simulink library "inp"  (Simulink 7.4)
settings: Solver=ode45  StartTime=0.0  StopTime=10.0  RelTol=1e-3
undefined symbols (not defined in the file): AINP_BrkPedalInterp_X_bar, C_TASK_10MS_S, ENUM_SHIFTER_D, ENUM_SHIFTER_N, ENUM_SHIFTER_P, ENUM_SHIFTER_R, KINP_BonnetCloseVehSpdThre_kph, KINP_EDUCoolantTempFilTm_s, KINP_EDUOilPressureFilTm_s, KINP_EDUOilTempFilTm_s, KINP_EDUSynchDisp_mm, KINP_EDUSynchPosnPWMDC_pct_LowerLimit, KINP_EDUSynchPosnPWMDC_pct_ovrdflg, KINP_EDUSynchPosnPWMDC_pct_ovrdval, KINP_EDUSynchPosnPWMDC_pct_UpperLimit, KINP_ShifterPosConfirmD_s, KINP_ShifterPosConfirmN_s, KINP_ShifterPosConfirmP_s, KINP_ShifterPosConfirmR_s, KINP_SingleAccPedalFltRateLim_pct, KINP_TMSpd2VehSpdSigNeg_rpm, KINP_TMSpd2VehSpdSigPos_rpm, KINP_ValidCheck_EDUSynchPosnPWMDC_dec, KINP_ValidCheck_EDUSynchPosnPWMDC_inc, KINP_ValidCheck_EDUSynchPosnPWMDC_lim, KINP_VehSpdSigKeepThres_kph, KPH2MPS, MIN2SEC, MINP_BrkPedalInterp_pct, MPS2KPH, PI, seat_version_control_block_callbacks, TIRE_RADIUS
libraries: inp_lib x166, hcu_lib x4, simulink x1
(part 5 of 9)

== system inp/INP/INP_10MS/Message (10ms) ABS_DSC_HSC_FrP03 ==
  BHAL_IN_10ms : Inport
  BSRV_In_ovrdflgs : Inport  Port=2
  BSRV_In_ovrdvals : Inport  Port=3
  VINP_DSCMsgAlive_flg : Inport  Port=4
  Bus Selector1 : BusSelector  OutputSignals=VHAL_BrakePressureValidIn_flg
  Bus Selector110 : BusSelector  OutputSignals=VSRV_BrakePressureIn_bar_ovrdflg
  Bus Selector112 : BusSelector  OutputSignals=VSRV_BrakePressureIn_bar_ovrdval
  Bus Selector25 : BusSelector  OutputSignals=VHAL_BrakePressureIn_bar
  Bus Selector4 : BusSelector  OutputSignals=VSRV_ABSDSCHSCFrP03Active_flg_ovrdflg
  Bus Selector8 : BusSelector  OutputSignals=VSRV_ABSDSCHSCFrP03Active_flg_ovrdval
  Subsys VINP_ABSDSCHSCFrP03Active_flg : inp_lib/override  SystemSampleTime=-1  cal_ovrdflg=KINP_ABSDSCHSCFrP03Active_ovrdflg  cal_ovrdval=KINP_ABSDSCHSCFrP03Active_flg_ovrdval
  Subsys VINP_BrkPedalPosn_pct : inp_lib/valid_msgactv_sat_ovrd  SystemSampleTime=-1  cal_ovrdflg=KINP_BrakePressure_bar_ovrdflg  cal_ovrdval=KINP_BrakePressure_bar_ovrdval  lim=KINP_ValidCheck_BrakePressure_lim  inc=KINP_ValidCheck_BrakePressure_inc  dec=KINP_ValidCheck_BrakePressure_dec  default=KINP_BrakePressureDefault_bar  hi=KINP_BrakePressure_bar_Max  lo=KINP_BrakePressure_bar_Min
  inputs_bus1 : BusCreator  Inputs=3
  lu1d_BrkPedalInterp : Lookup  InputValues=AINP_BrkPedalInterp_X_bar  Table=MINP_BrkPedalInterp_pct  LookUpMeth=Interpolation-Use End Values  OutDataType=sfix(16)  OutScaling=2^0
      settings: AttributesFormatString=input=%<inputvalues>\noutput=%<outputvalues>
  BINP_ABS_DSC_HSC_FrP03 : Outport  OutDataType=sfix(16)  OutScaling=2^0
  wires:
  [BSRV_In_ovrdvals] -> Bus Selector112/1
  [BSRV_In_ovrdflgs] -> Bus Selector110/1
  inputs_bus1/1 -> BINP_ABS_DSC_HSC_FrP03/1  "BINP_ABS_DSC_HSC_FrP03"
  BSRV_In_ovrdvals/1 -> [BSRV_In_ovrdvals]
  BSRV_In_ovrdflgs/1 -> [BSRV_In_ovrdflgs]
  VINP_DSCMsgAlive_flg/1 -> [VINP_DSCMsgAlive_flg]
  BHAL_IN_10ms/1 -> Bus Selector1/1, Bus Selector25/1
  [VINP_DSCMsgAlive_flg] -> [MsgAlive_flgs], Subsys VINP_ABSDSCHSCFrP03Active_flg/1  "VHAL_ABSDSCHSCFrP03Active_flg"
  [BSRV_In_ovrdflgs] -> Bus Selector4/1
  [BSRV_In_ovrdvals] -> Bus Selector8/1
  Bus Selector4/1 -> Subsys VINP_ABSDSCHSCFrP03Active_flg/2  "<VSRV_ABSDSCHSCFrP03Active_flg_ovrdflg>"
  Bus Selector8/1 -> Subsys VINP_ABSDSCHSCFrP03Active_flg/3  "<VSRV_ABSDSCHSCFrP03Active_flg_ovrdval>"
  Subsys VINP_ABSDSCHSCFrP03Active_flg/1 -> inputs_bus1/3  "VINP_ABSDSCHSCFrP03Active_flg"
  lu1d_BrkPedalInterp/1 -> inputs_bus1/1  "VINP_BrkPedalPosn_pct"
  Bus Selector25/1 -> Subsys VINP_BrkPedalPosn_pct/1  "<VHAL_BrakePressureIn_bar>"
  Bus Selector1/1 -> Subsys VINP_BrkPedalPosn_pct/2  "<VHAL_BrakePressureValidIn_flg>"
  Bus Selector110/1 -> Subsys VINP_BrkPedalPosn_pct/3  "<VSRV_BrakePressureIn_bar_ovrdflg>"
  Bus Selector112/1 -> Subsys VINP_BrkPedalPosn_pct/4  "<VSRV_BrakePressureIn_bar_ovrdval>"
  [MsgAlive_flgs] -> Subsys VINP_BrkPedalPosn_pct/5
  Subsys VINP_BrkPedalPosn_pct/1 -> lu1d_BrkPedalInterp/1  "VINP_BrakePressure_bar"
  Subsys VINP_BrkPedalPosn_pct/2 -> inputs_bus1/2  "VINP_BrkPedalPosnValid_flg"

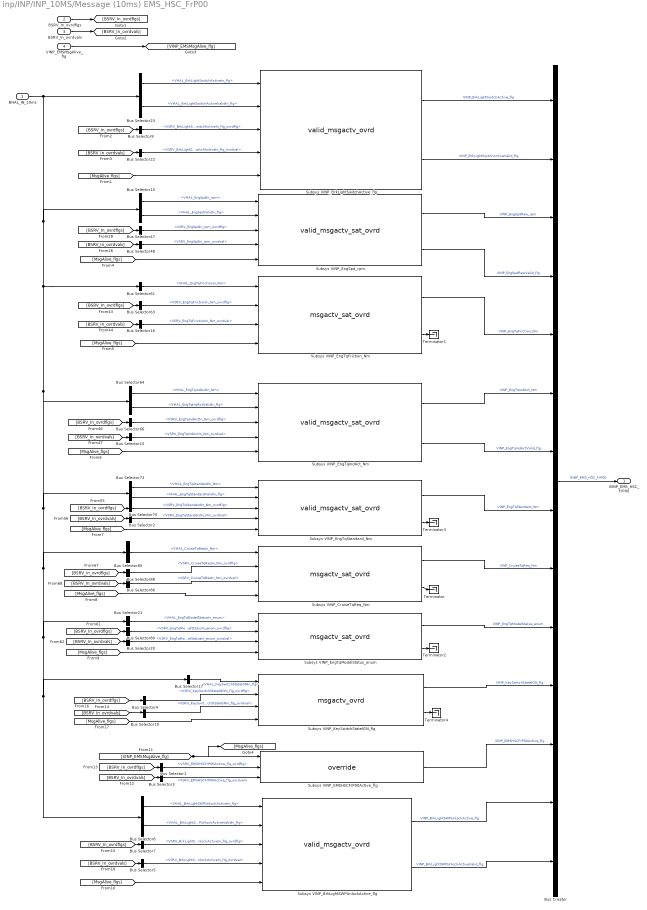
== system inp/INP/INP_10MS/Message (10ms) EMS_HSC_FrP00 ==
  BHAL_IN_10ms : Inport
  BSRV_In_ovrdflgs : Inport  Port=2
  BSRV_In_ovrdvals : Inport  Port=3
  VINP_EMSMsgAlive_flg : Inport  Port=4
  Bus Creator : BusCreator  Inputs=14
  Bus Selector1 : BusSelector  OutputSignals=VSRV_EMSHSCFrP00Active_flg_ovrdflg
  Bus Selector10 : BusSelector  OutputSignals=VHAL_EngSpdIn_rpm,VHAL_EngSpdValidIn_flg
  Bus Selector15 : BusSelector  OutputSignals=VSRV_EngTqIndActIn_Nm_ovrdval
  Bus Selector16 : BusSelector  OutputSignals=VSRV_EngTqFrictionIn_Nm_ovrdval
  Bus Selector17 : BusSelector  OutputSignals=VHAL_KeySwitchStateIGNIn_flg
  Bus Selector19 : BusSelector  OutputSignals=VSRV_KeySwitchStateIGNIn_flg_ovrdval
  Bus Selector2 : BusSelector  OutputSignals=VSRV_EngTqStandardIn_Nm_ovrdval
  Bus Selector20 : BusSelector  OutputSignals=VSRV_EngTqModelStatusIn_enum_ovrdval
  Bus Selector21 : BusSelector  OutputSignals=VHAL_EngTqModelStatusIn_enum
  Bus Selector22 : BusSelector  OutputSignals=VSRV_BrkLightSwitchActiveIn_flg_ovrdval
  Bus Selector23 : BusSelector  OutputSignals=VHAL_BrkLightSwitchActiveIn_flg,VHAL_BrkLightSwitchActiveValidIn_flg
  Bus Selector3 : BusSelector  OutputSignals=VSRV_EMSHSCFrP00Active_flg_ovrdval
  Bus Selector4 : BusSelector  OutputSignals=VSRV_KeySwitchStateIGNIn_flg_ovrdflg
  Bus Selector47 : BusSelector  OutputSignals=VSRV_EngSpdIn_rpm_ovrdflg
  Bus Selector48 : BusSelector  OutputSignals=VSRV_EngSpdIn_rpm_ovrdval
  Bus Selector5 : BusSelector  OutputSignals=VSRV_BrkLightSWPUnlockActiveIn_flg_ovrdval
  Bus Selector6 : BusSelector  OutputSignals=VHAL_BrkLightSWPUnlockActiveIn_flg,VHAL_BrkLightSWPUnlockActiveValidIn_flg
  Bus Selector61 : BusSelector  OutputSignals=VHAL_EngTqFrictionIn_Nm
  Bus Selector63 : BusSelector  OutputSignals=VSRV_EngTqFrictionIn_Nm_ovrdflg
  Bus Selector64 : BusSelector  OutputSignals=VHAL_EngTqIndActIn_Nm,VHAL_EngTqIndActValidIn_flg
  Bus Selector66 : BusSelector  OutputSignals=VSRV_EngTqIndActIn_Nm_ovrdflg
  Bus Selector7 : BusSelector  OutputSignals=VSRV_BrkLightSWPUnlockActiveIn_flg_ovrdflg
  Bus Selector73 : BusSelector  OutputSignals=VHAL_EngTqStandardIn_Nm,VHAL_EngTqStandardValidIn_flg
  Bus Selector75 : BusSelector  OutputSignals=VSRV_EngTqStandardIn_Nm_ovrdflg
  Bus Selector80 : BusSelector  OutputSignals=VSRV_EngTqModelStatusIn_enum_ovrdflg
  Bus Selector85 : BusSelector  OutputSignals=VHAL_CruiseTqReqIn_Nm
  Bus Selector86 : BusSelector  OutputSignals=VSRV_CruiseTqReqIn_Nm_ovrdval
  Bus Selector88 : BusSelector  OutputSignals=VSRV_CruiseTqReqIn_Nm_ovrdflg
  Bus Selector9 : BusSelector  OutputSignals=VSRV_BrkLightSwitchActiveIn_flg_ovrdflg
  Subsys VINP_BrkLightSWPUnlockActive_flg : inp_lib/valid_msgactv_ovrd  SystemSampleTime=-1  cal_ovrdflg=KINP_BrkLightSWPUnlockActive_flg_ovrdflg  cal_ovrdval=KINP_BrkLightSWPUnlockActive_flg_ovrdval  lim=KINP_ValidCheck_BrkLightSWPUnlockActive_lim  inc=KINP_ValidCheck_BrkLightSWPUnlockActive_inc  dec=KINP_ValidCheck_BrkLightSWPUnlockActive_dec  default=KINP_BrkLightSWPUnlockActiveDefault_flg
  Subsys VINP_BrkLightSwitchActive_flg : inp_lib/valid_msgactv_ovrd  SystemSampleTime=-1  cal_ovrdflg=KINP_BrkLightSwitchActive_flg_ovrdflg  cal_ovrdval=KINP_BrkLightSwitchActive_flg_ovrdval  lim=KINP_ValidCheck_BrkLightSwitchActive_lim  inc=KINP_ValidCheck_BrkLightSwitchActive_inc  dec=KINP_ValidCheck_BrkLightSwitchActive_dec  default=KINP_BrkLightSwitchActiveDefault_flg
  Subsys VINP_CruiseTqReq_Nm : inp_lib/msgactv_sat_ovrd  SystemSampleTime=-1  cal_ovrdflg=KINP_CruiseTqReq_Nm_ovrdflg  cal_ovrdval=KINP_CruiseTqReq_Nm_ovrdval  default=KINP_CruiseTqReqDefault_Nm  hi=KINP_CruiseTqReq_Nm_Max  lo=KINP_CruiseTqReq_Nm_Min
  Subsys VINP_EMSHSCFrP00Active_flg : inp_lib/override  SystemSampleTime=-1  cal_ovrdflg=KINP_EMSHSCFrP00Active_ovrdflg  cal_ovrdval=KINP_EMSHSCFrP00Active_flg_ovrdval
  Subsys VINP_EngSpd_rpm : inp_lib/valid_msgactv_sat_ovrd  SystemSampleTime=-1  cal_ovrdflg=KINP_EngSpd_rpm_ovrdflg  cal_ovrdval=KINP_EngSpd_rpm_ovrdval  lim=KINP_ValidCheck_EngSpd_lim  inc=KINP_ValidCheck_EngSpd_inc  dec=KINP_ValidCheck_EngSpd_dec  default=KINP_EngSpdDefault_rpm  hi=KINP_EngSpd_rpm_Max  lo=KINP_EngSpd_rpm_Min
  Subsys VINP_EngTqFriction_Nm : inp_lib/msgactv_sat_ovrd  SystemSampleTime=-1  cal_ovrdflg=KINP_EngTqFriction_Nm_ovrdflg  cal_ovrdval=KINP_EngTqFriction_Nm_ovrdval  default=KINP_EngTqFrictionDefault_Nm  hi=KINP_EngTqFriction_Nm_Max  lo=KINP_EngTqFriction_Nm_Min
  Subsys VINP_EngTqIndAct_Nm : inp_lib/valid_msgactv_sat_ovrd  SystemSampleTime=-1  cal_ovrdflg=KINP_EngTqIndAct_Nm_ovrdflg  cal_ovrdval=KINP_EngTqIndAct_Nm_ovrdval  lim=KINP_ValidCheck_EngTqIndAct_lim  inc=KINP_ValidCheck_EngTqIndAct_inc  dec=KINP_ValidCheck_EngTqIndAct_dec  default=KINP_EngTqIndActDefault_Nm  hi=KINP_EngTqIndAct_Nm_Max  lo=KINP_EngTqIndAct_Nm_Min
  Subsys VINP_EngTqModelStatus_enum : inp_lib/msgactv_sat_ovrd  SystemSampleTime=-1  cal_ovrdflg=KINP_EngTqModelStatus_enum_ovrdflg  cal_ovrdval=KINP_EngTqModelStatus_enum_ovrdval  default=KINP_EngTqModelStatusDefault_enum  hi=KINP_EngTqModelStatus_enum_Max  lo=KINP_EngTqModelStatus_enum_Min
  Subsys VINP_EngTqStandard_Nm : inp_lib/valid_msgactv_sat_ovrd  SystemSampleTime=-1  cal_ovrdflg=KINP_EngTqStandard_Nm_ovrdflg  cal_ovrdval=KINP_EngTqStandard_Nm_ovrdval  lim=KINP_ValidCheck_EngTqStandard_lim  inc=KINP_ValidCheck_EngTqStandard_inc  dec=KINP_ValidCheck_EngTqStandard_dec  default=KINP_EngTqStandardDefault_Nm  hi=KINP_EngTqStandard_Nm_Max  lo=KINP_EngTqStandard_Nm_Min
  Subsys VINP_KeySwitchStateIGN_flg : inp_lib/msgactv_ovrd  SystemSampleTime=-1  cal_ovrdflg=KINP_KeySwitchStateIGN_flg_ovrdflg  cal_ovrdval=KINP_KeySwitchStateIGN_flg_ovrdval  default=KINP_KeySwitchStateIGNDefault_flg
  Terminator{,1..4} (5 alike) : Terminator
  BINP_EMS_HSC_FrP00 : Outport  OutDataType=sfix(16)  OutScaling=2^0
  wires:
  Subsys VINP_BrkLightSwitchActive_flg/1 -> Bus Creator/1  "VINP_BrkLightSwitchActive_flg"
  Bus Selector9/1 -> Subsys VINP_BrkLightSwitchActive_flg/3  "<VSRV_BrkLightSwitchActiveIn_flg_ovrdflg>"
  Bus Selector6/2 -> Subsys VINP_BrkLightSWPUnlockActive_flg/2  "<VHAL_BrkLightSWPUnlockActiveValidIn_flg>"
  Bus Selector23/2 -> Subsys VINP_BrkLightSwitchActive_flg/2  "<VHAL_BrkLightSwitchActiveValidIn_flg>"
  [MsgAlive_flgs] -> Subsys VINP_BrkLightSwitchActive_flg/5
  Bus Selector22/1 -> Subsys VINP_BrkLightSwitchActive_flg/4  "<VSRV_BrkLightSwitchActiveIn_flg_ovrdval>"
  [VINP_EMSMsgAlive_flg] -> [MsgAlive_flgs], Subsys VINP_EMSHSCFrP00Active_flg/1
  [BSRV_In_ovrdflgs] -> Bus Selector1/1
  [BSRV_In_ovrdvals] -> Bus Selector3/1
  [BSRV_In_ovrdflgs] -> Bus Selector4/1
  [BSRV_In_ovrdvals] -> Bus Selector19/1
  VINP_EMSMsgAlive_flg/1 -> [VINP_EMSMsgAlive_flg]
  BSRV_In_ovrdflgs/1 -> [BSRV_In_ovrdflgs]
  BSRV_In_ovrdvals/1 -> [BSRV_In_ovrdvals]
  [BSRV_In_ovrdflgs] -> Bus Selector80/1
  [BSRV_In_ovrdvals] -> Bus Selector20/1
  Bus Creator/1 -> BINP_EMS_HSC_FrP00/1  "BINP_EMS_HSC_FrP00"
  [BSRV_In_ovrdflgs] -> Bus Selector9/1
  [BSRV_In_ovrdvals] -> Bus Selector22/1
  [BSRV_In_ovrdflgs] -> Bus Selector47/1
  [BSRV_In_ovrdvals] -> Bus Selector48/1
  [BSRV_In_ovrdflgs] -> Bus Selector63/1
  [BSRV_In_ovrdvals] -> Bus Selector16/1
  [BSRV_In_ovrdflgs] -> Bus Selector66/1
  [BSRV_In_ovrdvals] -> Bus Selector15/1
  [BSRV_In_ovrdflgs] -> Bus Selector75/1
  [BSRV_In_ovrdvals] -> Bus Selector2/1
  [BSRV_In_ovrdflgs] -> Bus Selector88/1
  [BSRV_In_ovrdvals] -> Bus Selector86/1
  BHAL_IN_10ms/1 -> Bus Selector61/1, Bus Selector64/1, Bus Selector73/1, Bus Selector85/1, Bus Selector21/1, Bus Selector17/1, Bus Selector6/1, Bus Selector10/1, Bus Selector23/1
  [BSRV_In_ovrdflgs] -> Bus Selector7/1
  [BSRV_In_ovrdvals] -> Bus Selector5/1
  Bus Selector6/1 -> Subsys VINP_BrkLightSWPUnlockActive_flg/1  "<VHAL_BrkLightSWPUnlockActiveIn_flg>"
  Bus Selector7/1 -> Subsys VINP_BrkLightSWPUnlockActive_flg/3  "<VSRV_BrkLightSWPUnlockActiveIn_flg_ovrdflg>"
  Bus Selector5/1 -> Subsys VINP_BrkLightSWPUnlockActive_flg/4  "<VSRV_BrkLightSWPUnlockActiveIn_flg_ovrdval>"
  [MsgAlive_flgs] -> Subsys VINP_BrkLightSWPUnlockActive_flg/5
  Subsys VINP_BrkLightSWPUnlockActive_flg/1 -> Bus Creator/13  "VINP_BrkLightSWPUnlockActive_flg"
  Subsys VINP_BrkLightSWPUnlockActive_flg/2 -> Bus Creator/14  "VINP_BrkLightSWPUnlockActiveValid_flg"
  Bus Selector23/1 -> Subsys VINP_BrkLightSwitchActive_flg/1  "<VHAL_BrkLightSwitchActiveIn_flg>"
  Subsys VINP_BrkLightSwitchActive_flg/2 -> Bus Creator/2  "VINP_BrkLightSwitchActiveValid_flg"
  Bus Selector85/1 -> Subsys VINP_CruiseTqReq_Nm/1  "<VHAL_CruiseTqReqIn_Nm>"
  Bus Selector88/1 -> Subsys VINP_CruiseTqReq_Nm/2  "<VSRV_CruiseTqReqIn_Nm_ovrdflg>"
  Bus Selector86/1 -> Subsys VINP_CruiseTqReq_Nm/3  "<VSRV_CruiseTqReqIn_Nm_ovrdval>"
  [MsgAlive_flgs] -> Subsys VINP_CruiseTqReq_Nm/4
  Subsys VINP_CruiseTqReq_Nm/1 -> Bus Creator/9  "VINP_CruiseTqReq_Nm"
  Subsys VINP_CruiseTqReq_Nm/2 -> Terminator/1
  Bus Selector1/1 -> Subsys VINP_EMSHSCFrP00Active_flg/2  "<VSRV_EMSHSCFrP00Active_flg_ovrdflg>"
  Bus Selector3/1 -> Subsys VINP_EMSHSCFrP00Active_flg/3  "<VSRV_EMSHSCFrP00Active_flg_ovrdval>"
  Subsys VINP_EMSHSCFrP00Active_flg/1 -> Bus Creator/12  "VINP_EMSHSCFrP00Active_flg"
  Bus Selector61/1 -> Subsys VINP_EngTqFriction_Nm/1  "<VHAL_EngTqFrictionIn_Nm>"
  Bus Selector63/1 -> Subsys VINP_EngTqFriction_Nm/2  "<VSRV_EngTqFrictionIn_Nm_ovrdflg>"
  Bus Selector16/1 -> Subsys VINP_EngTqFriction_Nm/3  "<VSRV_EngTqFrictionIn_Nm_ovrdval>"
  [MsgAlive_flgs] -> Subsys VINP_EngTqFriction_Nm/4
  Subsys VINP_EngTqFriction_Nm/1 -> Bus Creator/5  "VINP_EngTqFriction_Nm"
  Subsys VINP_EngTqFriction_Nm/2 -> Terminator1/1
  Bus Selector64/1 -> Subsys VINP_EngTqIndAct_Nm/1  "<VHAL_EngTqIndActIn_Nm>"
  Bus Selector64/2 -> Subsys VINP_EngTqIndAct_Nm/2  "<VHAL_EngTqIndActValidIn_flg>"
  Bus Selector66/1 -> Subsys VINP_EngTqIndAct_Nm/3  "<VSRV_EngTqIndActIn_Nm_ovrdflg>"
  Bus Selector15/1 -> Subsys VINP_EngTqIndAct_Nm/4  "<VSRV_EngTqIndActIn_Nm_ovrdval>"
  [MsgAlive_flgs] -> Subsys VINP_EngTqIndAct_Nm/5
  Subsys VINP_EngTqIndAct_Nm/1 -> Bus Creator/6  "VINP_EngTqIndAct_Nm"
  Subsys VINP_EngTqIndAct_Nm/2 -> Bus Creator/7  "VINP_EngTqIndActValid_flg"
  Bus Selector21/1 -> Subsys VINP_EngTqModelStatus_enum/1  "<VHAL_EngTqModelStatusIn_enum>"
  Bus Selector80/1 -> Subsys VINP_EngTqModelStatus_enum/2  "<VSRV_EngTqModelStatusIn_enum_ovrdflg>"
  Bus Selector20/1 -> Subsys VINP_EngTqModelStatus_enum/3  "<VSRV_EngTqModelStatusIn_enum_ovrdval>"
  [MsgAlive_flgs] -> Subsys VINP_EngTqModelStatus_enum/4
  Subsys VINP_EngTqModelStatus_enum/1 -> Bus Creator/10  "VINP_EngTqModelStatus_enum"
  Subsys VINP_EngTqModelStatus_enum/2 -> Terminator2/1
  Bus Selector73/1 -> Subsys VINP_EngTqStandard_Nm/1  "<VHAL_EngTqStandardIn_Nm>"
  Bus Selector73/2 -> Subsys VINP_EngTqStandard_Nm/2  "<VHAL_EngTqStandardValidIn_flg>"
  Bus Selector75/1 -> Subsys VINP_EngTqStandard_Nm/3  "<VSRV_EngTqStandardIn_Nm_ovrdflg>"
  Bus Selector2/1 -> Subsys VINP_EngTqStandard_Nm/4  "<VSRV_EngTqStandardIn_Nm_ovrdval>"
  [MsgAlive_flgs] -> Subsys VINP_EngTqStandard_Nm/5
  Subsys VINP_EngTqStandard_Nm/1 -> Bus Creator/8  "VINP_EngTqStandard_Nm"
  Subsys VINP_EngTqStandard_Nm/2 -> Terminator3/1
  Bus Selector17/1 -> Subsys VINP_KeySwitchStateIGN_flg/1  "<VHAL_KeySwitchStateIGNIn_flg>"
  Bus Selector4/1 -> Subsys VINP_KeySwitchStateIGN_flg/2  "<VSRV_KeySwitchStateIGNIn_flg_ovrdflg>"
  Bus Selector19/1 -> Subsys VINP_KeySwitchStateIGN_flg/3  "<VSRV_KeySwitchStateIGNIn_flg_ovrdval>"
  [MsgAlive_flgs] -> Subsys VINP_KeySwitchStateIGN_flg/4
  Subsys VINP_KeySwitchStateIGN_flg/1 -> Bus Creator/11  "VINP_KeySwitchStateIGN_flg"
  Subsys VINP_KeySwitchStateIGN_flg/2 -> Terminator4/1
  Bus Selector10/1 -> Subsys VINP_EngSpd_rpm/1  "<VHAL_EngSpdIn_rpm>"
  Bus Selector10/2 -> Subsys VINP_EngSpd_rpm/2  "<VHAL_EngSpdValidIn_flg>"
  Bus Selector47/1 -> Subsys VINP_EngSpd_rpm/3  "<VSRV_EngSpdIn_rpm_ovrdflg>"
  Bus Selector48/1 -> Subsys VINP_EngSpd_rpm/4  "<VSRV_EngSpdIn_rpm_ovrdval>"
  [MsgAlive_flgs] -> Subsys VINP_EngSpd_rpm/5
  Subsys VINP_EngSpd_rpm/1 -> Bus Creator/3  "VINP_EngSpdRaw_rpm"
  Subsys VINP_EngSpd_rpm/2 -> Bus Creator/4  "VINP_EngSpdRawValid_flg"

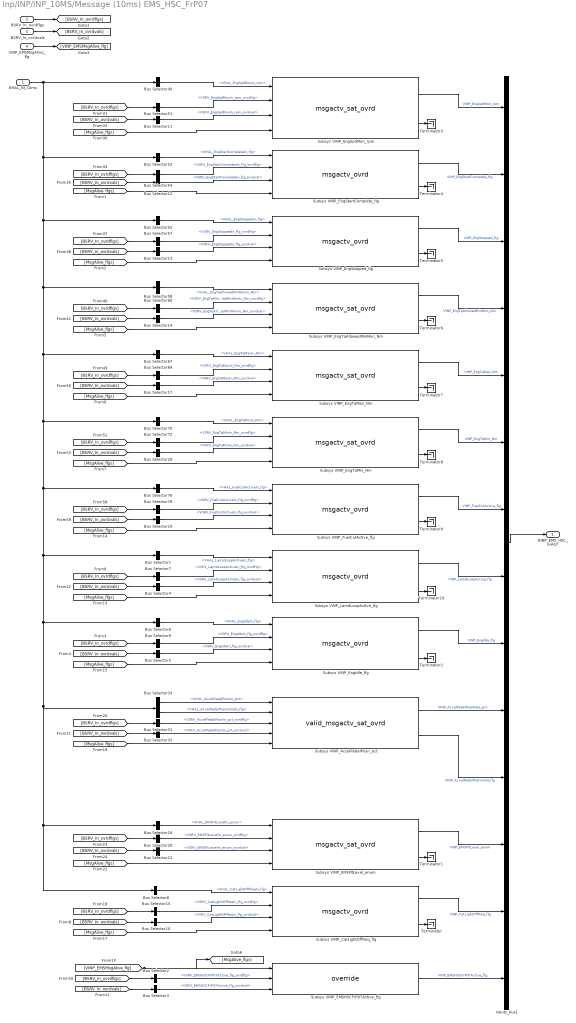
== system inp/INP/INP_10MS/Message (10ms) EMS_HSC_FrP07 ==
  BHAL_IN_10ms : Inport
  BSRV_In_ovrdflgs : Inport  Port=2
  BSRV_In_ovrdvals : Inport  Port=3
  VINP_EMSMsgAlive_flg : Inport  Port=4
  Bus Selector1 : BusSelector  OutputSignals=VHAL_LamdLoopActiveIn_flg
  Bus Selector10 : BusSelector  OutputSignals=VSRV_CatLightOffReqIn_flg_ovrdval
  Bus Selector11 : BusSelector  OutputSignals=VSRV_EngSpdMonIn_rpm_ovrdval
  Bus Selector12 : BusSelector  OutputSignals=VSRV_EngStartCompleteIn_flg_ovrdval
  Bus Selector13 : BusSelector  OutputSignals=VSRV_EngStoppedIn_flg_ovrdval
  Bus Selector14 : BusSelector  OutputSignals=VSRV_EngTqAllowedMinMonIn_Nm_ovrdval
  Bus Selector15 : BusSelector  OutputSignals=VSRV_CatLightOffReqIn_flg_ovrdflg
  Bus Selector16 : BusSelector  OutputSignals=VHAL_EMSFltLevelIn_enum
  Bus Selector17 : BusSelector  OutputSignals=VSRV_EngTqMaxIn_Nm_ovrdval
  Bus Selector18 : BusSelector  OutputSignals=VSRV_EngTqMinIn_Nm_ovrdval
  Bus Selector19 : BusSelector  OutputSignals=VSRV_FuelCutActiveIn_flg_ovrdval
  Bus Selector2 : BusSelector  OutputSignals=VSRV_EMSHSCFrP07Active_flg_ovrdflg
  Bus Selector20 : BusSelector  OutputSignals=VSRV_EMSFltLevelIn_enum_ovrdflg
  Bus Selector21 : BusSelector  OutputSignals=VSRV_EMSFltLevelIn_enum_ovrdval
  Bus Selector3 : BusSelector  OutputSignals=VSRV_EMSHSCFrP07Active_flg_ovrdval
  Bus Selector31 : BusSelector  OutputSignals=VSRV_AccelPedalPosnIn_pct_ovrdflg
  Bus Selector32 : BusSelector  OutputSignals=VSRV_AccelPedalPosnIn_pct_ovrdval
  Bus Selector33 : BusSelector  OutputSignals=VHAL_AccelPedalPosnIn_pct,VHAL_AccelPedalPosnValidIn_flg
  Bus Selector4 : BusSelector  OutputSignals=VSRV_LamdLoopActiveIn_flg_ovrdval
  Bus Selector49 : BusSelector  OutputSignals=VHAL_EngSpdMonIn_rpm
  Bus Selector5 : BusSelector  OutputSignals=VSRV_EngIdleIn_flg_ovrdval
  Bus Selector51 : BusSelector  OutputSignals=VSRV_EngSpdMonIn_rpm_ovrdflg
  Bus Selector52 : BusSelector  OutputSignals=VHAL_EngStartCompleteIn_flg
  Bus Selector54 : BusSelector  OutputSignals=VSRV_EngStartCompleteIn_flg_ovrdflg
  Bus Selector55 : BusSelector  OutputSignals=VHAL_EngStoppedIn_flg
  Bus Selector57 : BusSelector  OutputSignals=VSRV_EngStoppedIn_flg_ovrdflg
  Bus Selector58 : BusSelector  OutputSignals=VHAL_EngTqAllowedMinMonIn_Nm
  Bus Selector6 : BusSelector  OutputSignals=VHAL_EngIdleIn_flg
  Bus Selector60 : BusSelector  OutputSignals=VSRV_EngTqAllowedMinMonIn_Nm_ovrdflg
  Bus Selector67 : BusSelector  OutputSignals=VHAL_EngTqMaxIn_Nm
  Bus Selector69 : BusSelector  OutputSignals=VSRV_EngTqMaxIn_Nm_ovrdflg
  Bus Selector7 : BusSelector  OutputSignals=VSRV_LamdLoopActiveIn_flg_ovrdflg
  Bus Selector70 : BusSelector  OutputSignals=VHAL_EngTqMinIn_Nm
  Bus Selector72 : BusSelector  OutputSignals=VSRV_EngTqMinIn_Nm_ovrdflg
  Bus Selector76 : BusSelector  OutputSignals=VHAL_FuelCutActiveIn_flg
  Bus Selector78 : BusSelector  OutputSignals=VSRV_FuelCutActiveIn_flg_ovrdflg
  Bus Selector8 : BusSelector  OutputSignals=VHAL_CatLightOffReqIn_flg
  Bus Selector9 : BusSelector  OutputSignals=VSRV_EngIdleIn_flg_ovrdflg
  Subsys VINP_AccelPedalPosn_pct : inp_lib/valid_msgactv_sat_ovrd  SystemSampleTime=-1  cal_ovrdflg=KINP_AccelPedalPosn_pct_ovrdflg  cal_ovrdval=KINP_AccelPedalPosn_pct_ovrdval  lim=KINP_ValidCheck_AccelPedalPosn_lim  inc=KINP_ValidCheck_AccelPedalPosn_inc  dec=KINP_ValidCheck_AccelPedalPosn_dec  default=KINP_AccelPedalPosnDefault_pct  hi=KINP_AccelPedalPosn_pct_Max  lo=KINP_AccelPedalPosn_pct_Min
  Subsys VINP_CatLightOffReq_flg : inp_lib/msgactv_ovrd  SystemSampleTime=-1  cal_ovrdflg=KINP_CatLightOffReq_flg_ovrdflg  cal_ovrdval=KINP_CatLightOffReq_flg_ovrdval  default=KINP_CatLightOffReqDefault_flg
  Subsys VINP_EMSFltLevel_enum : inp_lib/msgactv_sat_ovrd  SystemSampleTime=-1  cal_ovrdflg=KINP_EMSFltLevel_enum_ovrdflg  cal_ovrdval=KINP_EMSFltLevel_enum_ovrdval  default=KINP_EMSFltLevelDefault_enum  hi=KINP_EMSFltLevel_enum_Max  lo=KINP_EMSFltLevel_enum_Min
  Subsys VINP_EMSHSCFrP07Active_flg : inp_lib/override  SystemSampleTime=-1  cal_ovrdflg=KINP_EMSHSCFrP07Active_ovrdflg  cal_ovrdval=KINP_EMSHSCFrP07Active_flg_ovrdval
  Subsys VINP_EngIdle_flg : inp_lib/msgactv_ovrd  SystemSampleTime=-1  cal_ovrdflg=KINP_EngIdle_flg_ovrdflg  cal_ovrdval=KINP_EngIdle_flg_ovrdval  default=KINP_EngIdleDefault_flg
  Subsys VINP_EngSpdMon_rpm : inp_lib/msgactv_sat_ovrd  SystemSampleTime=-1  cal_ovrdflg=KINP_EngSpdMon_rpm_ovrdflg  cal_ovrdval=KINP_EngSpdMon_rpm_ovrdval  default=KINP_EngSpdMonDefault_rpm  hi=KINP_EngSpdMon_rpm_Max  lo=KINP_EngSpdMon_rpm_Min
  Subsys VINP_EngStartComplete_flg : inp_lib/msgactv_ovrd  SystemSampleTime=-1  cal_ovrdflg=KINP_EngStartComplete_flg_ovrdflg  cal_ovrdval=KINP_EngStartComplete_flg_ovrdval  default=KINP_EngStartCompleteDefault_flg
  Subsys VINP_EngStopped_flg : inp_lib/msgactv_ovrd  SystemSampleTime=-1  cal_ovrdflg=KINP_EngStopped_flg_ovrdflg  cal_ovrdval=KINP_EngStopped_flg_ovrdval  default=KINP_EngStoppedDefault_flg
  Subsys VINP_EngTqAllowedMinMon_Nm : inp_lib/msgactv_sat_ovrd  SystemSampleTime=-1  cal_ovrdflg=KINP_EngTqAllowedMinMon_Nm_ovrdflg  cal_ovrdval=KINP_EngTqAllowedMinMon_Nm_ovrdval  default=KINP_EngTqAllowedMinMonDefault_Nm  hi=KINP_EngTqAllowedMinMon_Nm_Max  lo=KINP_EngTqAllowedMinMon_Nm_Min
  Subsys VINP_EngTqMax_Nm : inp_lib/msgactv_sat_ovrd  SystemSampleTime=-1  cal_ovrdflg=KINP_EngTqMax_Nm_ovrdflg  cal_ovrdval=KINP_EngTqMax_Nm_ovrdval  default=KINP_EngTqMaxDefault_Nm  hi=KINP_EngTqMax_Nm_Max  lo=KINP_EngTqMax_Nm_Min
  Subsys VINP_EngTqMin_Nm : inp_lib/msgactv_sat_ovrd  SystemSampleTime=-1  cal_ovrdflg=KINP_EngTqMin_Nm_ovrdflg  cal_ovrdval=KINP_EngTqMin_Nm_ovrdval  default=KINP_EngTqMinDefault_Nm  hi=KINP_EngTqMin_Nm_Max  lo=KINP_EngTqMin_Nm_Min
  Subsys VINP_FuelCutActive_flg : inp_lib/msgactv_ovrd  SystemSampleTime=-1  cal_ovrdflg=KINP_FuelCutActive_flg_ovrdflg  cal_ovrdval=KINP_FuelCutActive_flg_ovrdval  default=KINP_FuelCutActiveDefault_flg
  Subsys VINP_LamdLoopActive_flg : inp_lib/msgactv_ovrd  SystemSampleTime=-1  cal_ovrdflg=KINP_LamdLoopActive_flg_ovrdflg  cal_ovrdval=KINP_LamdLoopActive_flg_ovrdval  default=KINP_LamdLoopActiveDefault_flg
  Terminator{,1..10} (11 alike) : Terminator
  inputs_bus1 : BusCreator  Inputs=14
  BINP_EMS_HSC_FrP07 : Outport  OutDataType=sfix(16)  OutScaling=2^0
  wires:
  [BSRV_In_ovrdflgs] -> Bus Selector20/1
  [BSRV_In_ovrdvals] -> Bus Selector21/1
  [BSRV_In_ovrdvals] -> Bus Selector3/1
  [BSRV_In_ovrdflgs] -> Bus Selector2/1
  [VINP_EMSMsgAlive_flg] -> [MsgAlive_flgs], Subsys VINP_EMSHSCFrP07Active_flg/1
  [BSRV_In_ovrdflgs] -> Bus Selector15/1
  [BSRV_In_ovrdvals] -> Bus Selector10/1
  [BSRV_In_ovrdvals] -> Bus Selector13/1
  [BSRV_In_ovrdflgs] -> Bus Selector57/1
  [BSRV_In_ovrdvals] -> Bus Selector5/1
  [BSRV_In_ovrdflgs] -> Bus Selector9/1
  [BSRV_In_ovrdvals] -> Bus Selector19/1
  [BSRV_In_ovrdflgs] -> Bus Selector78/1
  [BSRV_In_ovrdvals] -> Bus Selector18/1
  [BSRV_In_ovrdflgs] -> Bus Selector72/1
  [BSRV_In_ovrdvals] -> Bus Selector17/1
  [BSRV_In_ovrdflgs] -> Bus Selector69/1
  [BSRV_In_ovrdvals] -> Bus Selector14/1
  [BSRV_In_ovrdflgs] -> Bus Selector60/1
  [BSRV_In_ovrdvals] -> Bus Selector12/1
  [BSRV_In_ovrdflgs] -> Bus Selector54/1
  [BSRV_In_ovrdvals] -> Bus Selector11/1
  [BSRV_In_ovrdflgs] -> Bus Selector51/1
  BHAL_IN_10ms/1 -> Bus Selector16/1, Bus Selector8/1, Bus Selector33/1, Bus Selector6/1, Bus Selector1/1, Bus Selector76/1, Bus Selector70/1, Bus Selector67/1, Bus Selector58/1, Bus Selector55/1, Bus Selector52/1, Bus Selector49/1
  VINP_EMSMsgAlive_flg/1 -> [VINP_EMSMsgAlive_flg]
  BSRV_In_ovrdflgs/1 -> [BSRV_In_ovrdflgs]
  BSRV_In_ovrdvals/1 -> [BSRV_In_ovrdvals]
  [BSRV_In_ovrdflgs] -> Bus Selector7/1
  [BSRV_In_ovrdvals] -> Bus Selector4/1
  [BSRV_In_ovrdvals] -> Bus Selector32/1
  [BSRV_In_ovrdflgs] -> Bus Selector31/1
  inputs_bus1/1 -> BINP_EMS_HSC_FrP07/1
  Bus Selector8/1 -> Subsys VINP_CatLightOffReq_flg/1  "<VHAL_CatLightOffReqIn_flg>"
  Bus Selector15/1 -> Subsys VINP_CatLightOffReq_flg/2  "<VSRV_CatLightOffReqIn_flg_ovrdflg>"
  Bus Selector10/1 -> Subsys VINP_CatLightOffReq_flg/3  "<VSRV_CatLightOffReqIn_flg_ovrdval>"
  [MsgAlive_flgs] -> Subsys VINP_CatLightOffReq_flg/4
  Subsys VINP_CatLightOffReq_flg/1 -> inputs_bus1/13  "VINP_CatLightOffReq_flg"
  Subsys VINP_CatLightOffReq_flg/2 -> Terminator/1
  Bus Selector16/1 -> Subsys VINP_EMSFltLevel_enum/1  "<VHAL_EMSFltLevelIn_enum>"
  Bus Selector20/1 -> Subsys VINP_EMSFltLevel_enum/2  "<VSRV_EMSFltLevelIn_enum_ovrdflg>"
  Bus Selector21/1 -> Subsys VINP_EMSFltLevel_enum/3  "<VSRV_EMSFltLevelIn_enum_ovrdval>"
  [MsgAlive_flgs] -> Subsys VINP_EMSFltLevel_enum/4
  Subsys VINP_EMSFltLevel_enum/1 -> inputs_bus1/12  "VINP_EMSFltLevel_enum"
  Subsys VINP_EMSFltLevel_enum/2 -> Terminator1/1
  Bus Selector2/1 -> Subsys VINP_EMSHSCFrP07Active_flg/2  "<VSRV_EMSHSCFrP07Active_flg_ovrdflg>"
  Bus Selector3/1 -> Subsys VINP_EMSHSCFrP07Active_flg/3  "<VSRV_EMSHSCFrP07Active_flg_ovrdval>"
  Subsys VINP_EMSHSCFrP07Active_flg/1 -> inputs_bus1/14  "VINP_EMSHSCFrP07Active_flg"
  Bus Selector6/1 -> Subsys VINP_EngIdle_flg/1  "<VHAL_EngIdleIn_flg>"
  Bus Selector9/1 -> Subsys VINP_EngIdle_flg/2  "<VSRV_EngIdleIn_flg_ovrdflg>"
  Bus Selector5/1 -> Subsys VINP_EngIdle_flg/3  "<VSRV_EngIdleIn_flg_ovrdval>"
  [MsgAlive_flgs] -> Subsys VINP_EngIdle_flg/4
  Subsys VINP_EngIdle_flg/1 -> inputs_bus1/9  "VINP_EngIdle_flg"
  Subsys VINP_EngIdle_flg/2 -> Terminator2/1
  Bus Selector49/1 -> Subsys VINP_EngSpdMon_rpm/1  "<VHAL_EngSpdMonIn_rpm>"
  Bus Selector51/1 -> Subsys VINP_EngSpdMon_rpm/2  "<VSRV_EngSpdMonIn_rpm_ovrdflg>"
  Bus Selector11/1 -> Subsys VINP_EngSpdMon_rpm/3  "<VSRV_EngSpdMonIn_rpm_ovrdval>"
  [MsgAlive_flgs] -> Subsys VINP_EngSpdMon_rpm/4
  Subsys VINP_EngSpdMon_rpm/1 -> inputs_bus1/1  "VINP_EngSpdMon_rpm"
  Subsys VINP_EngSpdMon_rpm/2 -> Terminator3/1
  Bus Selector52/1 -> Subsys VINP_EngStartComplete_flg/1  "<VHAL_EngStartCompleteIn_flg>"
  Bus Selector54/1 -> Subsys VINP_EngStartComplete_flg/2  "<VSRV_EngStartCompleteIn_flg_ovrdflg>"
  Bus Selector12/1 -> Subsys VINP_EngStartComplete_flg/3  "<VSRV_EngStartCompleteIn_flg_ovrdval>"
  [MsgAlive_flgs] -> Subsys VINP_EngStartComplete_flg/4
  Subsys VINP_EngStartComplete_flg/1 -> inputs_bus1/2  "VINP_EngStartComplete_flg"
  Subsys VINP_EngStartComplete_flg/2 -> Terminator4/1
  Bus Selector55/1 -> Subsys VINP_EngStopped_flg/1  "<VHAL_EngStoppedIn_flg>"
  Bus Selector57/1 -> Subsys VINP_EngStopped_flg/2  "<VSRV_EngStoppedIn_flg_ovrdflg>"
  Bus Selector13/1 -> Subsys VINP_EngStopped_flg/3  "<VSRV_EngStoppedIn_flg_ovrdval>"
  [MsgAlive_flgs] -> Subsys VINP_EngStopped_flg/4
  Subsys VINP_EngStopped_flg/1 -> inputs_bus1/3  "VINP_EngStopped_flg"
  Subsys VINP_EngStopped_flg/2 -> Terminator5/1
  Bus Selector58/1 -> Subsys VINP_EngTqAllowedMinMon_Nm/1  "<VHAL_EngTqAllowedMinMonIn_Nm>"
  Bus Selector60/1 -> Subsys VINP_EngTqAllowedMinMon_Nm/2  "<VSRV_EngTqAllowedMinMonIn_Nm_ovrdflg>"
  Bus Selector14/1 -> Subsys VINP_EngTqAllowedMinMon_Nm/3  "<VSRV_EngTqAllowedMinMonIn_Nm_ovrdval>"
  [MsgAlive_flgs] -> Subsys VINP_EngTqAllowedMinMon_Nm/4
  Subsys VINP_EngTqAllowedMinMon_Nm/1 -> inputs_bus1/4  "VINP_EngTqAllowedMinMon_Nm"
  Subsys VINP_EngTqAllowedMinMon_Nm/2 -> Terminator6/1
  Bus Selector67/1 -> Subsys VINP_EngTqMax_Nm/1  "<VHAL_EngTqMaxIn_Nm>"
  Bus Selector69/1 -> Subsys VINP_EngTqMax_Nm/2  "<VSRV_EngTqMaxIn_Nm_ovrdflg>"
  Bus Selector17/1 -> Subsys VINP_EngTqMax_Nm/3  "<VSRV_EngTqMaxIn_Nm_ovrdval>"
  [MsgAlive_flgs] -> Subsys VINP_EngTqMax_Nm/4
  Subsys VINP_EngTqMax_Nm/1 -> inputs_bus1/5  "VINP_EngTqMax_Nm"
  Subsys VINP_EngTqMax_Nm/2 -> Terminator7/1
  Bus Selector70/1 -> Subsys VINP_EngTqMin_Nm/1  "<VHAL_EngTqMinIn_Nm>"
  Bus Selector72/1 -> Subsys VINP_EngTqMin_Nm/2  "<VSRV_EngTqMinIn_Nm_ovrdflg>"
  Bus Selector18/1 -> Subsys VINP_EngTqMin_Nm/3  "<VSRV_EngTqMinIn_Nm_ovrdval>"
  [MsgAlive_flgs] -> Subsys VINP_EngTqMin_Nm/4
  Subsys VINP_EngTqMin_Nm/1 -> inputs_bus1/6  "VINP_EngTqMin_Nm"
  Subsys VINP_EngTqMin_Nm/2 -> Terminator8/1
  Bus Selector76/1 -> Subsys VINP_FuelCutActive_flg/1  "<VHAL_FuelCutActiveIn_flg>"
  Bus Selector78/1 -> Subsys VINP_FuelCutActive_flg/2  "<VSRV_FuelCutActiveIn_flg_ovrdflg>"
  Bus Selector19/1 -> Subsys VINP_FuelCutActive_flg/3  "<VSRV_FuelCutActiveIn_flg_ovrdval>"
  [MsgAlive_flgs] -> Subsys VINP_FuelCutActive_flg/4
  Subsys VINP_FuelCutActive_flg/1 -> inputs_bus1/7  "VINP_FuelCutActive_flg"
  Subsys VINP_FuelCutActive_flg/2 -> Terminator9/1
  Bus Selector1/1 -> Subsys VINP_LamdLoopActive_flg/1  "<VHAL_LamdLoopActiveIn_flg>"
  Bus Selector7/1 -> Subsys VINP_LamdLoopActive_flg/2  "<VSRV_LamdLoopActiveIn_flg_ovrdflg>"
  Bus Selector4/1 -> Subsys VINP_LamdLoopActive_flg/3  "<VSRV_LamdLoopActiveIn_flg_ovrdval>"
  [MsgAlive_flgs] -> Subsys VINP_LamdLoopActive_flg/4
  Subsys VINP_LamdLoopActive_flg/1 -> inputs_bus1/8  "VINP_LamdLoopActive_flg"
  Subsys VINP_LamdLoopActive_flg/2 -> Terminator10/1
  Bus Selector33/1 -> Subsys VINP_AccelPedalPosn_pct/1  "<VHAL_AccelPedalPosnIn_pct>"
  Bus Selector33/2 -> Subsys VINP_AccelPedalPosn_pct/2  "<VHAL_AccelPedalPosnValidIn_flg>"
  Bus Selector31/1 -> Subsys VINP_AccelPedalPosn_pct/3  "<VSRV_AccelPedalPosnIn_pct_ovrdflg>"
  Bus Selector32/1 -> Subsys VINP_AccelPedalPosn_pct/4  "<VSRV_AccelPedalPosnIn_pct_ovrdval>"
  [MsgAlive_flgs] -> Subsys VINP_AccelPedalPosn_pct/5
  Subsys VINP_AccelPedalPosn_pct/1 -> inputs_bus1/10  "VINP_AccelPedalPosnRaw_pct"
  Subsys VINP_AccelPedalPosn_pct/2 -> inputs_bus1/11  "VINP_AccelPedalPosnValid_flg"

== system inp/INP/INP_10MS/Message (10ms) ISC_HSC2_FrP03 ==
  BHAL_IN_10ms : Inport
  BSRV_In_ovrdflgs : Inport  Port=2
  BSRV_In_ovrdvals : Inport  Port=3
  VINP_ISCMsgAlive_flg : Inport  Port=4
  Bus Creator : BusCreator  Inputs=8
  Bus Selector1 : BusSelector  OutputSignals=VSRV_ISGDiagReqIn_flg_ovrdval
  Bus Selector103 : BusSelector  OutputSignals=VHAL_ISGTqActIn_Nm
  Bus Selector104 : BusSelector  OutputSignals=VSRV_ISGTqActIn_Nm_ovrdflg
  Bus Selector16 : BusSelector  OutputSignals=VSRV_ISGACShortCircReadyIn_flg_ovrdflg
  Bus Selector17 : BusSelector  OutputSignals=VHAL_ISGACShortCircReadyIn_flg
  Bus Selector18 : BusSelector  OutputSignals=VHAL_ISGSpdIn_rpm
  Bus Selector19 : BusSelector  OutputSignals=VSRV_ISGACShortCircReadyIn_flg_ovrdval
  Bus Selector2 : BusSelector  OutputSignals=VSRV_ISCHSC2FrP03Active_flg_ovrdflg
  Bus Selector23 : BusSelector  OutputSignals=VSRV_ISGTqActIn_Nm_ovrdval
  Bus Selector3 : BusSelector  OutputSignals=VSRV_ISCHSC2FrP03Active_flg_ovrdval
  Bus Selector4 : BusSelector  OutputSignals=VHAL_ISGSpdValidIn_flg
  Bus Selector5 : BusSelector  OutputSignals=VHAL_ISGTqActValidIn_flg
  Bus Selector56 : BusSelector  OutputSignals=VHAL_ISGModeIn_enum
  Bus Selector57 : BusSelector  OutputSignals=VSRV_ISGModeIn_enum_ovrdflg
  Bus Selector6 : BusSelector  OutputSignals=VHAL_ISGDiagReqIn_flg
  Bus Selector7 : BusSelector  OutputSignals=VSRV_ISGDiagReqIn_flg_ovrdflg
  Bus Selector8 : BusSelector  OutputSignals=VSRV_ISGModeIn_enum_ovrdval
  Bus Selector86 : BusSelector  OutputSignals=VSRV_ISGSpdIn_rpm_ovrdflg
  Bus Selector87 : BusSelector  OutputSignals=VSRV_ISGSpdIn_rpm_ovrdval
  Subsys VINP_ISCHSC2FrP03Active_flg : inp_lib/override  SystemSampleTime=-1  cal_ovrdflg=KINP_ISCHSC2FrP03Active_ovrdflg  cal_ovrdval=KINP_ISCHSC2FrP03Active_flg_ovrdval
  Subsys VINP_ISGACShortCircReady_flg : inp_lib/msgactv_ovrd  SystemSampleTime=-1  cal_ovrdflg=KINP_ISGACShortCircReady_flg_ovrdflg  cal_ovrdval=KINP_ISGACShortCircReady_flg_ovrdval  default=KINP_ISGACShortCircReadyDefault_flg
  Subsys VINP_ISGDiagReq_flg : inp_lib/msgactv_ovrd  SystemSampleTime=-1  cal_ovrdflg=KINP_ISGDiagReq_flg_ovrdflg  cal_ovrdval=KINP_ISGDiagReq_flg_ovrdval  default=KINP_ISGDiagReqDefault_flg
  Subsys VINP_ISGMode_enum : inp_lib/msgactv_sat_ovrd  SystemSampleTime=-1  cal_ovrdflg=KINP_ISGMode_enum_ovrdflg  cal_ovrdval=KINP_ISGMode_enum_ovrdval  default=KINP_ISGModeDefault_enum  hi=KINP_ISGMode_enum_Max  lo=KINP_ISGMode_enum_Min
  Subsys VINP_ISGSpeed_rpm : inp_lib/valid_msgactv_sat_ovrd  SystemSampleTime=-1  cal_ovrdflg=KINP_ISGSpd_rpm_ovrdflg  cal_ovrdval=KINP_ISGSpd_rpm_ovrdval  lim=KINP_ValidCheck_ISGSpd_lim  inc=KINP_ValidCheck_ISGSpd_inc  dec=KINP_ValidCheck_ISGSpd_dec  default=KINP_ISGSpdDefault_rpm  hi=KINP_ISGSpd_rpm_Max  lo=KINP_ISGSpd_rpm_Min
  Subsys VINP_ISGTqAct_Nm : inp_lib/valid_msgactv_sat_ovrd  SystemSampleTime=-1  cal_ovrdflg=KINP_ISGTqAct_Nm_ovrdflg  cal_ovrdval=KINP_ISGTqAct_Nm_ovrdval  lim=KINP_ValidCheck_ISGTqAct_lim  inc=KINP_ValidCheck_ISGTqAct_inc  dec=KINP_ValidCheck_ISGTqAct_dec  default=KINP_ISGTqActDefault_Nm  hi=KINP_ISGTqAct_Nm_Max  lo=KINP_ISGTqAct_Nm_Min
  Terminator : Terminator
  Terminator1 : Terminator
  Terminator2 : Terminator
  BINP_ISC_HSC2_FrP03 : Outport
  wires:
  Bus Creator/1 -> BINP_ISC_HSC2_FrP03/1  "BINP_ISC_HSC2_FrP03"
  BSRV_In_ovrdvals/1 -> [BSRV_In_ovrdvals]
  BSRV_In_ovrdflgs/1 -> [BSRV_In_ovrdflgs]
  VINP_ISCMsgAlive_flg/1 -> [VINP_ISCMsgAlive_flg]
  [BSRV_In_ovrdflgs] -> Bus Selector16/1
  [BSRV_In_ovrdvals] -> Bus Selector19/1
  BHAL_IN_10ms/1 -> Bus Selector6/1, Bus Selector56/1, Bus Selector18/1, Bus Selector4/1, Bus Selector103/1, Bus Selector5/1, Bus Selector17/1
  [VINP_ISCMsgAlive_flg] -> [MsgAlive_flgs], Subsys VINP_ISCHSC2FrP03Active_flg/1  "VHAL_ISCHSC2FrP03Active_flg"
  [BSRV_In_ovrdflgs] -> Bus Selector2/1
  [BSRV_In_ovrdvals] -> Bus Selector3/1
  [BSRV_In_ovrdflgs] -> Bus Selector7/1
  [BSRV_In_ovrdvals] -> Bus Selector1/1
  [BSRV_In_ovrdvals] -> Bus Selector23/1
  [BSRV_In_ovrdflgs] -> Bus Selector104/1
  [BSRV_In_ovrdvals] -> Bus Selector87/1
  [BSRV_In_ovrdflgs] -> Bus Selector86/1
  [BSRV_In_ovrdflgs] -> Bus Selector57/1
  [BSRV_In_ovrdvals] -> Bus Selector8/1
  Bus Selector2/1 -> Subsys VINP_ISCHSC2FrP03Active_flg/2  "<VSRV_ISCHSC2FrP03Active_flg_ovrdflg>"
  Bus Selector3/1 -> Subsys VINP_ISCHSC2FrP03Active_flg/3  "<VSRV_ISCHSC2FrP03Active_flg_ovrdval>"
  Subsys VINP_ISCHSC2FrP03Active_flg/1 -> Bus Creator/8  "VINP_ISCHSC2FrP03Active_flg"
  Bus Selector17/1 -> Subsys VINP_ISGACShortCircReady_flg/1  "<VHAL_ISGACShortCircReadyIn_flg>"
  Bus Selector16/1 -> Subsys VINP_ISGACShortCircReady_flg/2  "<VSRV_ISGACShortCircReadyIn_flg_ovrdflg>"
  Bus Selector19/1 -> Subsys VINP_ISGACShortCircReady_flg/3  "<VSRV_ISGACShortCircReadyIn_flg_ovrdval>"
  [MsgAlive_flgs] -> Subsys VINP_ISGACShortCircReady_flg/4
  Subsys VINP_ISGACShortCircReady_flg/1 -> Bus Creator/1  "VINP_ISGACShortCircReady_flg"
  Subsys VINP_ISGACShortCircReady_flg/2 -> Terminator/1
  Bus Selector6/1 -> Subsys VINP_ISGDiagReq_flg/1  "<VHAL_ISGDiagReqIn_flg>"
  Bus Selector7/1 -> Subsys VINP_ISGDiagReq_flg/2  "<VSRV_ISGDiagReqIn_flg_ovrdflg>"
  Bus Selector1/1 -> Subsys VINP_ISGDiagReq_flg/3  "<VSRV_ISGDiagReqIn_flg_ovrdval>"
  [MsgAlive_flgs] -> Subsys VINP_ISGDiagReq_flg/4
  Subsys VINP_ISGDiagReq_flg/1 -> Bus Creator/2  "VINP_ISGDiagReq_flg"
  Subsys VINP_ISGDiagReq_flg/2 -> Terminator1/1
  Bus Selector56/1 -> Subsys VINP_ISGMode_enum/1  "<VHAL_ISGModeIn_enum>"
  Bus Selector57/1 -> Subsys VINP_ISGMode_enum/2  "<VSRV_ISGModeIn_enum_ovrdflg>"
  Bus Selector8/1 -> Subsys VINP_ISGMode_enum/3  "<VSRV_ISGModeIn_enum_ovrdval>"
  [MsgAlive_flgs] -> Subsys VINP_ISGMode_enum/4
  Subsys VINP_ISGMode_enum/1 -> Bus Creator/3  "VINP_ISGMode_enum"
  Subsys VINP_ISGMode_enum/2 -> Terminator2/1
  Bus Selector103/1 -> Subsys VINP_ISGTqAct_Nm/1  "<VHAL_ISGTqActIn_Nm>"
  Bus Selector5/1 -> Subsys VINP_ISGTqAct_Nm/2  "<VHAL_ISGTqActValidIn_flg>"
  Bus Selector104/1 -> Subsys VINP_ISGTqAct_Nm/3  "<VSRV_ISGTqActIn_Nm_ovrdflg>"
  Bus Selector23/1 -> Subsys VINP_ISGTqAct_Nm/4  "<VSRV_ISGTqActIn_Nm_ovrdval>"
  [MsgAlive_flgs] -> Subsys VINP_ISGTqAct_Nm/5
  Subsys VINP_ISGTqAct_Nm/1 -> Bus Creator/6  "VINP_ISGTqAct_Nm"
  Subsys VINP_ISGTqAct_Nm/2 -> Bus Creator/7  "VINP_ISGTqActValid_flg"
  Bus Selector18/1 -> Subsys VINP_ISGSpeed_rpm/1  "<VHAL_ISGSpdIn_rpm>"
  Bus Selector4/1 -> Subsys VINP_ISGSpeed_rpm/2  "<VHAL_ISGSpdValidIn_flg>"
  Bus Selector86/1 -> Subsys VINP_ISGSpeed_rpm/3  "<VSRV_ISGSpdIn_rpm_ovrdflg>"
  Bus Selector87/1 -> Subsys VINP_ISGSpeed_rpm/4  "<VSRV_ISGSpdIn_rpm_ovrdval>"
  [MsgAlive_flgs] -> Subsys VINP_ISGSpeed_rpm/5
  Subsys VINP_ISGSpeed_rpm/1 -> Bus Creator/4  "VINP_ISGSpdRaw_rpm"
  Subsys VINP_ISGSpeed_rpm/2 -> Bus Creator/5  "VINP_ISGSpdRawValid_flg"

== system inp/INP/INP_10MS/Message (10ms) ISC_HSC2_FrP04 ==
  BHAL_IN_10ms : Inport
  BSRV_In_ovrdflgs : Inport  Port=2
  BSRV_In_ovrdvals : Inport  Port=3
  VINP_ISCMsgAlive_flg : Inport  Port=4
  Bus Creator : BusCreator  Inputs=5
  Bus Selector1 : BusSelector  OutputSignals=VHAL_ISGInvtCurrIn_A
  Bus Selector106 : BusSelector  OutputSignals=VHAL_ISGTqAvailMinIn_Nm
  Bus Selector107 : BusSelector  OutputSignals=VSRV_ISGTqAvailMinIn_Nm_ovrdflg
  Bus Selector109 : BusSelector  OutputSignals=VSRV_ISGTqAvailMinIn_Nm_ovrdval
  Bus Selector110 : BusSelector  OutputSignals=VSRV_ISGTqAvailMaxIn_Nm_ovrdflg
  Bus Selector112 : BusSelector  OutputSignals=VSRV_ISGTqAvailMaxIn_Nm_ovrdval
  Bus Selector15 : BusSelector  OutputSignals=VHAL_ISGSurgeDampActiveIn_flg
  Bus Selector16 : BusSelector  OutputSignals=VSRV_ISGSurgeDampActiveIn_flg_ovrdflg
  Bus Selector2 : BusSelector  OutputSignals=VSRV_ISCHSC2FrP04Active_flg_ovrdflg
  Bus Selector25 : BusSelector  OutputSignals=VHAL_ISGTqAvailMaxIn_Nm
  Bus Selector3 : BusSelector  OutputSignals=VSRV_ISCHSC2FrP04Active_flg_ovrdval
  Bus Selector4 : BusSelector  OutputSignals=VHAL_ISGTqAvailMaxValidIn_flg
  Bus Selector5 : BusSelector  OutputSignals=VHAL_ISGTqAvailMinValidIn_flg
  Bus Selector6 : BusSelector  OutputSignals=VSRV_ISGInvtCurrIn_A_ovrdflg
  Bus Selector7 : BusSelector  OutputSignals=VSRV_ISGInvtCurrIn_A_ovrdval
  Bus Selector8 : BusSelector  OutputSignals=VHAL_ISGInvtCurrValidIn_flg
  Bus Selector9 : BusSelector  OutputSignals=VSRV_ISGSurgeDampActiveIn_flg_ovrdval
  Subsys VINP_ISCHSC2FrP04Active_flg : inp_lib/override  SystemSampleTime=-1  cal_ovrdflg=KINP_ISCHSC2FrP04Active_ovrdflg  cal_ovrdval=KINP_ISCHSC2FrP04Active_flg_ovrdval
  Subsys VINP_ISGInvtCurr_A : inp_lib/valid_msgactv_sat_ovrd  SystemSampleTime=-1  cal_ovrdflg=KINP_ISGInvtCurr_A_ovrdflg  cal_ovrdval=KINP_ISGInvtCurr_A_ovrdval  lim=KINP_ValidCheck_ISGInvtCurr_lim  inc=KINP_ValidCheck_ISGInvtCurr_inc  dec=KINP_ValidCheck_ISGInvtCurr_dec  default=KINP_ISGInvtCurrDefault_A  hi=KINP_ISGInvtCurr_A_Max  lo=KINP_ISGInvtCurr_A_Min
  Subsys VINP_ISGSurgeDampActive_flg : inp_lib/msgactv_ovrd  SystemSampleTime=-1  cal_ovrdflg=KINP_ISGSurgeDampActive_flg_ovrdflg  cal_ovrdval=KINP_ISGSurgeDampActive_flg_ovrdval  default=KINP_ISGSurgeDampActiveDefault_flg
  Subsys VINP_ISGTqAvailMax_Nm : inp_lib/valid_msgactv_sat_ovrd  SystemSampleTime=-1  cal_ovrdflg=KINP_ISGTqAvailMax_Nm_ovrdflg  cal_ovrdval=KINP_ISGTqAvailMax_Nm_ovrdval  lim=KINP_ValidCheck_ISGTqAvailMax_lim  inc=KINP_ValidCheck_ISGTqAvailMax_inc  dec=KINP_ValidCheck_ISGTqAvailMax_dec  default=KINP_ISGTqAvailMaxDefault_Nm  hi=KINP_ISGTqAvailMax_Nm_Max  lo=KINP_ISGTqAvailMax_Nm_Min
  Subsys VINP_ISGTqAvailMin_Nm : inp_lib/valid_msgactv_sat_ovrd  SystemSampleTime=-1  cal_ovrdflg=KINP_ISGTqAvailMin_Nm_ovrdflg  cal_ovrdval=KINP_ISGTqAvailMin_Nm_ovrdval  lim=KINP_ValidCheck_ISGTqAvailMin_lim  inc=KINP_ValidCheck_ISGTqAvailMin_inc  dec=KINP_ValidCheck_ISGTqAvailMin_dec  default=KINP_ISGTqAvailMinDefault_Nm  hi=KINP_ISGTqAvailMin_Nm_Max  lo=KINP_ISGTqAvailMin_Nm_Min
  Terminator{,1..3} (4 alike) : Terminator
  BINP_ISC_HSC2_FrP04 : Outport
  wires:
  [BSRV_In_ovrdflgs] -> Bus Selector6/1
  [BSRV_In_ovrdvals] -> Bus Selector7/1
  [VINP_ISCMsgAlive_flg] -> [MsgAlive_flgs], Subsys VINP_ISCHSC2FrP04Active_flg/1  "VHAL_ISCHSC2FrP04Active_flg"
  [BSRV_In_ovrdflgs] -> Bus Selector2/1
  [BSRV_In_ovrdvals] -> Bus Selector3/1
  [BSRV_In_ovrdvals] -> Bus Selector112/1
  [BSRV_In_ovrdflgs] -> Bus Selector110/1
  Bus Creator/1 -> BINP_ISC_HSC2_FrP04/1  "BINP_ISC_HSC2_FrP04"
  BSRV_In_ovrdvals/1 -> [BSRV_In_ovrdvals]
  BSRV_In_ovrdflgs/1 -> [BSRV_In_ovrdflgs]
  BHAL_IN_10ms/1 -> Bus Selector25/1, Bus Selector106/1, Bus Selector8/1, Bus Selector1/1, Bus Selector15/1, Bus Selector5/1, Bus Selector4/1
  VINP_ISCMsgAlive_flg/1 -> [VINP_ISCMsgAlive_flg]
  [BSRV_In_ovrdflgs] -> Bus Selector16/1
  [BSRV_In_ovrdvals] -> Bus Selector9/1
  [BSRV_In_ovrdflgs] -> Bus Selector107/1
  [BSRV_In_ovrdvals] -> Bus Selector109/1
  Bus Selector2/1 -> Subsys VINP_ISCHSC2FrP04Active_flg/2  "<VSRV_ISCHSC2FrP04Active_flg_ovrdflg>"
  Bus Selector3/1 -> Subsys VINP_ISCHSC2FrP04Active_flg/3  "<VSRV_ISCHSC2FrP04Active_flg_ovrdval>"
  Subsys VINP_ISCHSC2FrP04Active_flg/1 -> Bus Creator/5  "VINP_ISCHSC2FrP04Active_flg"
  Bus Selector1/1 -> Subsys VINP_ISGInvtCurr_A/1  "<VHAL_ISGInvtCurrIn_A>"
  Bus Selector8/1 -> Subsys VINP_ISGInvtCurr_A/2  "<VHAL_ISGInvtCurrValidIn_flg>"
  Bus Selector6/1 -> Subsys VINP_ISGInvtCurr_A/3  "<VSRV_ISGInvtCurrIn_A_ovrdflg>"
  Bus Selector7/1 -> Subsys VINP_ISGInvtCurr_A/4  "<VSRV_ISGInvtCurrIn_A_ovrdval>"
  [MsgAlive_flgs] -> Subsys VINP_ISGInvtCurr_A/5
  Subsys VINP_ISGInvtCurr_A/1 -> Bus Creator/4  "VINP_ISGInvtCurr_A"
  Subsys VINP_ISGInvtCurr_A/2 -> Terminator/1
  Bus Selector15/1 -> Subsys VINP_ISGSurgeDampActive_flg/1  "<VHAL_ISGSurgeDampActiveIn_flg>"
  Bus Selector16/1 -> Subsys VINP_ISGSurgeDampActive_flg/2  "<VSRV_ISGSurgeDampActiveIn_flg_ovrdflg>"
  Bus Selector9/1 -> Subsys VINP_ISGSurgeDampActive_flg/3  "<VSRV_ISGSurgeDampActiveIn_flg_ovrdval>"
  [MsgAlive_flgs] -> Subsys VINP_ISGSurgeDampActive_flg/4
  Subsys VINP_ISGSurgeDampActive_flg/1 -> Bus Creator/3  "VINP_ISGSurgeDampActive_flg"
  Subsys VINP_ISGSurgeDampActive_flg/2 -> Terminator1/1
  Bus Selector25/1 -> Subsys VINP_ISGTqAvailMax_Nm/1  "<VHAL_ISGTqAvailMaxIn_Nm>"
  Bus Selector4/1 -> Subsys VINP_ISGTqAvailMax_Nm/2  "<VHAL_ISGTqAvailMaxValidIn_flg>"
  Bus Selector110/1 -> Subsys VINP_ISGTqAvailMax_Nm/3  "<VSRV_ISGTqAvailMaxIn_Nm_ovrdflg>"
  Bus Selector112/1 -> Subsys VINP_ISGTqAvailMax_Nm/4  "<VSRV_ISGTqAvailMaxIn_Nm_ovrdval>"
  [MsgAlive_flgs] -> Subsys VINP_ISGTqAvailMax_Nm/5
  Subsys VINP_ISGTqAvailMax_Nm/1 -> Bus Creator/1  "VINP_ISGTqAvailMax_Nm"
  Subsys VINP_ISGTqAvailMax_Nm/2 -> Terminator2/1
  Bus Selector106/1 -> Subsys VINP_ISGTqAvailMin_Nm/1  "<VHAL_ISGTqAvailMinIn_Nm>"
  Bus Selector5/1 -> Subsys VINP_ISGTqAvailMin_Nm/2  "<VHAL_ISGTqAvailMinValidIn_flg>"
  Bus Selector107/1 -> Subsys VINP_ISGTqAvailMin_Nm/3  "<VSRV_ISGTqAvailMinIn_Nm_ovrdflg>"
  Bus Selector109/1 -> Subsys VINP_ISGTqAvailMin_Nm/4  "<VSRV_ISGTqAvailMinIn_Nm_ovrdval>"
  [MsgAlive_flgs] -> Subsys VINP_ISGTqAvailMin_Nm/5
  Subsys VINP_ISGTqAvailMin_Nm/1 -> Bus Creator/2  "VINP_ISGTqAvailMin_Nm"
  Subsys VINP_ISGTqAvailMin_Nm/2 -> Terminator3/1

== system inp/INP/INP_10MS/Message (10ms) SCU_HSC_FrP00 ==
  BHAL_IN_10ms : Inport
  BSRV_In_ovrdflgs : Inport  Port=2
  BSRV_In_ovrdvals : Inport  Port=3
  VINP_SCUMsgAlive_flg : Inport  Port=4
  Bus Selector1 : BusSelector  OutputSignals=VHAL_ShifterPosIn_enum,VHAL_ShifterPosValidIn_flg
  Bus Selector11 : BusSelector  OutputSignals=VSRV_ShifterInitIn_flg_ovrdflg
  Bus Selector12 : BusSelector  OutputSignals=VSRV_ShifterInitIn_flg_ovrdval
  Bus Selector2 : BusSelector  OutputSignals=VSRV_ShifterPosIn_enum_ovrdflg
  Bus Selector29 : BusSelector  OutputSignals=VHAL_ShifterFailIn_flg
  Bus Selector3 : BusSelector  OutputSignals=VSRV_ShifterPosIn_enum_ovrdval
  Bus Selector30 : BusSelector  OutputSignals=VSRV_ShifterFailIn_flg_ovrdflg
  Bus Selector31 : BusSelector  OutputSignals=VSRV_ShifterFailIn_flg_ovrdval
  Bus Selector4 : BusSelector  OutputSignals=VSRV_SCUHSCFrP00Active_flg_ovrdflg
  Bus Selector5 : BusSelector  OutputSignals=VSRV_ShifterPosProtFault_flg_ovrdflg
  Bus Selector6 : BusSelector  OutputSignals=VSRV_ShifterPosProtFault_flg_ovrdval
  Bus Selector7 : BusSelector  OutputSignals=VHAL_ShifterPosProtFaultIn_flg
  Bus Selector8 : BusSelector  OutputSignals=VSRV_SCUHSCFrP00Active_flg_ovrdval
  Bus Selector9 : BusSelector  OutputSignals=VHAL_ShifterInitIn_flg
  Subsys VINP_SCUHSCFrP00Active_flg : inp_lib/override  SystemSampleTime=-1  cal_ovrdflg=KINP_SCUHSCFrP00Active_ovrdflg  cal_ovrdval=KINP_SCUHSCFrP00Active_flg_ovrdval
  Subsys VINP_ShifterFail_flg : inp_lib/msgactv_ovrd  SystemSampleTime=-1  cal_ovrdflg=KINP_ShifterFail_flg_ovrdflg  cal_ovrdval=KINP_ShifterFail_flg_ovrdval  default=KINP_ShifterFailDefault_flg
  Subsys VINP_ShifterInit_flg : inp_lib/msgactv_ovrd  SystemSampleTime=-1  cal_ovrdflg=KINP_ShifterInit_flg_ovrdflg  cal_ovrdval=KINP_ShifterInit_flg_ovrdval  default=KINP_ShifterInitDefault_flg
  Subsys VINP_ShifterPosProtFault_flg : inp_lib/msgactv_ovrd  SystemSampleTime=-1  cal_ovrdflg=KINP_ShifterPosProtFault_flg_ovrdflg  cal_ovrdval=KINP_ShifterPosProtFault_flg_ovrdval  default=KINP_ShifterPosProtFaultDefault_flg
  Subsys VINP_ShifterPos_enum : inp_lib/valid_msgactv_sat_ovrd  SystemSampleTime=-1  cal_ovrdflg=KINP_ShifterPos_enum_ovrdflg  cal_ovrdval=KINP_ShifterPos_enum_ovrdval  lim=KINP_ValidCheck_ShifterPos_lim  inc=KINP_ValidCheck_ShifterPos_inc  dec=KINP_ValidCheck_ShifterPos_dec  default=KINP_ShifterPosDefault_enum  hi=KINP_ShifterPos_enum_Max  lo=KINP_ShifterPos_enum_Min
  Subsystem : Subsystem
  Terminator : Terminator
  Terminator1 : Terminator
  Terminator2 : Terminator
  inputs_bus1 : BusCreator  Inputs=6
  BINP_SCU_HSC_FrP00 : Outport  OutDataType=sfix(16)  OutScaling=2^0
  wires:
  [BSRV_In_ovrdvals] -> Bus Selector12/1
  [BSRV_In_ovrdflgs] -> Bus Selector11/1
  [VINP_SCUMsgAlive_flg] -> [MsgAlive_flgs], Subsys VINP_SCUHSCFrP00Active_flg/1
  [BSRV_In_ovrdflgs] -> Bus Selector4/1
  [BSRV_In_ovrdvals] -> Bus Selector8/1
  inputs_bus1/1 -> BINP_SCU_HSC_FrP00/1  "BINP_SCU_HSC_FrP00"
  BSRV_In_ovrdvals/1 -> [BSRV_In_ovrdvals]
  BSRV_In_ovrdflgs/1 -> [BSRV_In_ovrdflgs]
  VINP_SCUMsgAlive_flg/1 -> [VINP_SCUMsgAlive_flg]
  BHAL_IN_10ms/1 -> Bus Selector1/1, Bus Selector9/1, Bus Selector7/1, Bus Selector29/1
  [BSRV_In_ovrdflgs] -> Bus Selector30/1
  [BSRV_In_ovrdvals] -> Bus Selector31/1
  [BSRV_In_ovrdflgs] -> Bus Selector2/1
  [BSRV_In_ovrdvals] -> Bus Selector3/1
  [BSRV_In_ovrdvals] -> Bus Selector6/1
  [BSRV_In_ovrdflgs] -> Bus Selector5/1
  Bus Selector4/1 -> Subsys VINP_SCUHSCFrP00Active_flg/2  "<VSRV_SCUHSCFrP00Active_flg_ovrdflg>"
  Bus Selector8/1 -> Subsys VINP_SCUHSCFrP00Active_flg/3  "<VSRV_SCUHSCFrP00Active_flg_ovrdval>"
  Subsys VINP_SCUHSCFrP00Active_flg/1 -> inputs_bus1/6  "VINP_SCUHSCFrP00Active_flg"
  Bus Selector29/1 -> Subsys VINP_ShifterFail_flg/1  "<VHAL_ShifterFailIn_flg>"
  Bus Selector30/1 -> Subsys VINP_ShifterFail_flg/2  "<VSRV_ShifterFailIn_flg_ovrdflg>"
  Bus Selector31/1 -> Subsys VINP_ShifterFail_flg/3  "<VSRV_ShifterFailIn_flg_ovrdval>"
  [MsgAlive_flgs] -> Subsys VINP_ShifterFail_flg/4
  Subsys VINP_ShifterFail_flg/1 -> inputs_bus1/1  "VINP_ShifterFail_flg"
  Subsys VINP_ShifterFail_flg/2 -> Terminator/1
  Bus Selector9/1 -> Subsys VINP_ShifterInit_flg/1  "<VHAL_ShifterInitIn_flg>"
  Bus Selector11/1 -> Subsys VINP_ShifterInit_flg/2  "<VSRV_ShifterInitIn_flg_ovrdflg>"
  Bus Selector12/1 -> Subsys VINP_ShifterInit_flg/3  "<VSRV_ShifterInitIn_flg_ovrdval>"
  [MsgAlive_flgs] -> Subsys VINP_ShifterInit_flg/4
  Subsys VINP_ShifterInit_flg/1 -> inputs_bus1/4  "VINP_ShifterInit_flg"
  Subsys VINP_ShifterInit_flg/2 -> Terminator1/1
  Subsystem/1(VINP_ShifterPos_enum) -> inputs_bus1/2  "VINP_ShifterPos_enum"
  Bus Selector1/1 -> Subsys VINP_ShifterPos_enum/1  "<VHAL_ShifterPosIn_enum>"
  Bus Selector1/2 -> Subsys VINP_ShifterPos_enum/2  "<VHAL_ShifterPosValidIn_flg>"
  Bus Selector2/1 -> Subsys VINP_ShifterPos_enum/3  "<VSRV_ShifterPosIn_enum_ovrdflg>"
  Bus Selector3/1 -> Subsys VINP_ShifterPos_enum/4  "<VSRV_ShifterPosIn_enum_ovrdval>"
  [MsgAlive_flgs] -> Subsys VINP_ShifterPos_enum/5
  Subsys VINP_ShifterPos_enum/1 -> Subsystem/1(VINP_ShifterPosRaw_enum)  "VINP_ShifterPosRaw_enum"
  Subsys VINP_ShifterPos_enum/2 -> inputs_bus1/3  "VINP_ShifterPosValid_flg"
  Bus Selector7/1 -> Subsys VINP_ShifterPosProtFault_flg/1  "<VHAL_ShifterPosProtFaultIn_flg>"
  Bus Selector5/1 -> Subsys VINP_ShifterPosProtFault_flg/2  "<VSRV_ShifterPosProtFault_flg_ovrdflg>"
  Bus Selector6/1 -> Subsys VINP_ShifterPosProtFault_flg/3  "<VSRV_ShifterPosProtFault_flg_ovrdval>"
  [MsgAlive_flgs] -> Subsys VINP_ShifterPosProtFault_flg/4
  Subsys VINP_ShifterPosProtFault_flg/1 -> inputs_bus1/5  "VINP_ShifterPosProtFault_flg"
  Subsys VINP_ShifterPosProtFault_flg/2 -> Terminator2/1
